simulink model "SingleTank"  (Simulink 9.3)
settings: Solver=ode5  StartTime=0.0  StopTime=1000  FixedStep=1  MaxStep=0.1  RelTol=1e-3
StopFcn:
  | %plot_sim_data
Description:
  | The model describes dynamic properties of tank level system. The differential equation is:
  |                                            d/dt{Ah(t))=ku(t)-a*sqrt(2*g*h(t))
settings Model: Creator=Huynh Thai Hoang  LastModifiedBy=forev  ExtModeTrigMode=oneshot  ExtModeArmWhenConnect=off
settings SolverCC: InitialStep=0.1
settings DataIOCC: SaveOutput=off  SaveTime=off  SignalLoggingName=sigsOut
settings OptimizationCC: BooleanDataType=off  ExpressionDepthLimit=2147483647
settings DebuggingCC: SaveWithParameterizedLinksMsg=none  SignalResolutionControl=TryResolveAllWithWarning  MultiTaskDSMMsg=warning  MultiTaskCondExecSysMsg=none  StateNameClashWarn=warning
settings HardwareCC: TargetUnknown=on
settings GRTTargetCC: GeneratePreprocessorConditionals=Disable all

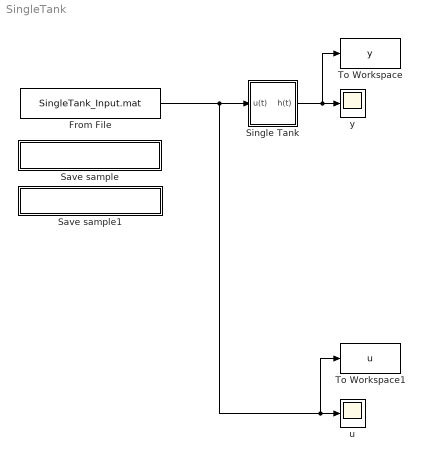
== system SingleTank ==
  From File : FromFile  FileName=SingleTank_Input.mat  SampleTime=0
  Save sample : Subsystem
      settings: OpenFcn=save_sample
      mask Display: disp('Save sampled data')
  Save sample1 : Subsystem
      settings: OpenFcn=signal_gen
      mask Display: disp('Generate Random Input')
  Single Tank : Subsystem  mask{A_min=100, A_max=200, a_out=1, h_max=100, k=60, U_max=12, C=0.8}
      mask prompts: A_min "Minimum cross area (cm2)"; A_max "Maximum cross area (cm2)"; a_out "Outlet area (cm2)"; h_max "Tank height (cm)"; k "Maximum pump flow (cm3/sec)"; U_max "Maximum control voltage (V)"; C "Discharge constant"
      mask init:
      | g=981;
      mask Display:
      | plot([0.1 0.3 0.9],[0.9 0.1 0.1]);
      | plot([0.9 0.7 0.9],[0.9 0.2 0.2]);
  To Workspace : ToWorkspace  VariableName=y  SampleTime=-1
  To Workspace1 : ToWorkspace  VariableName=u  SampleTime=-1
  u : Scope
  y : Scope
  wires:
  Single Tank/1(h(t)) -> To Workspace/1, y/1
  From File/1 -> Single Tank/1(u(t)), To Workspace1/1, u/1

== system SingleTank/Save sample ==

== system SingleTank/Save sample1 ==

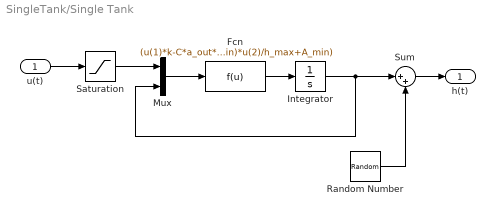
== system SingleTank/Single Tank ==
  u(t) : Inport
  Fcn : Fcn  Expr=(u(1)*k-C*a_out*sqrt(2*g*u(2)))/((A_max-A_min)*u(2)/h_max+A_min)
  Integrator : Integrator  LimitOutput=on  UpperSaturationLimit=h_max  LowerSaturationLimit=0
  Mux : Mux  Inputs=2
  Random Number : RandomNumber  Variance=0.1  SampleTime=0
  Saturation : Saturate  UpperLimit=12  LowerLimit=0
  Sum : Sum  Inputs=|++  SaturateOnIntegerOverflow=on
  h(t) : Outport
  wires:
  u(t)/1 -> Saturation/1
  Mux/1 -> Fcn/1
  Fcn/1 -> Integrator/1
  Integrator/1 -> Mux/2, Sum/1
  Saturation/1 -> Mux/1
  Sum/1 -> h(t)/1
  Random Number/1 -> Sum/2
